simulink model "EnergyEstimationCorrection"  (R2020a)
settings: Solver=FixedStepAuto  StartTime=0  StopTime=time.Time(length(time.Time))  FixedStep=0.10  MaxStep=0.04  RelTol=1e-3
model workspace (MAT data in the model file):
  displayStatus = 1
values from neighbouring files (symbols this model uses):
  routeInfo = 4011    [EnergyEstimationMain.m]
  trip = tripUpdate    [EnergyEstimationMain.m]
undefined symbols (not defined in the file or in its folder): EbatRoute, EdriveRoute, energyDriveActual, energyDriveTrip, energyDriveTripCurrent, eState, massEstimate, sRoute, start, startRoute, stop, stopRoute, timeRoute, vehicleInfo, y, y_Estimate
libraries: simulink x1
(part 1 of 2)
settings Model: Creator=20184719  LastModifiedBy=20184719
settings OptimizationCC: ZeroExternalMemoryAtStartup=off  ZeroInternalMemoryAtStartup=off
settings DebuggingCC: UnderSpecifiedDimensionMsg=warning
settings HardwareCC: ProdBitPerPointer=32  ProdBitPerSizeT=32  ProdBitPerPtrDiffT=32  ProdLargestAtomicInteger=Long  ProdWordSize=32  ProdHWDeviceType=ARM Compatible->ARM 10
settings RTWCC: GenCodeOnly=on  TargetLang=C++
settings GRTTargetCC: TargetLangStandard=C++03 (ISO)  MatFileLogging=off  MultiInstanceERTCode=on  CodeInterfacePackaging=C++ class  MultiInstanceErrorCode=Warning

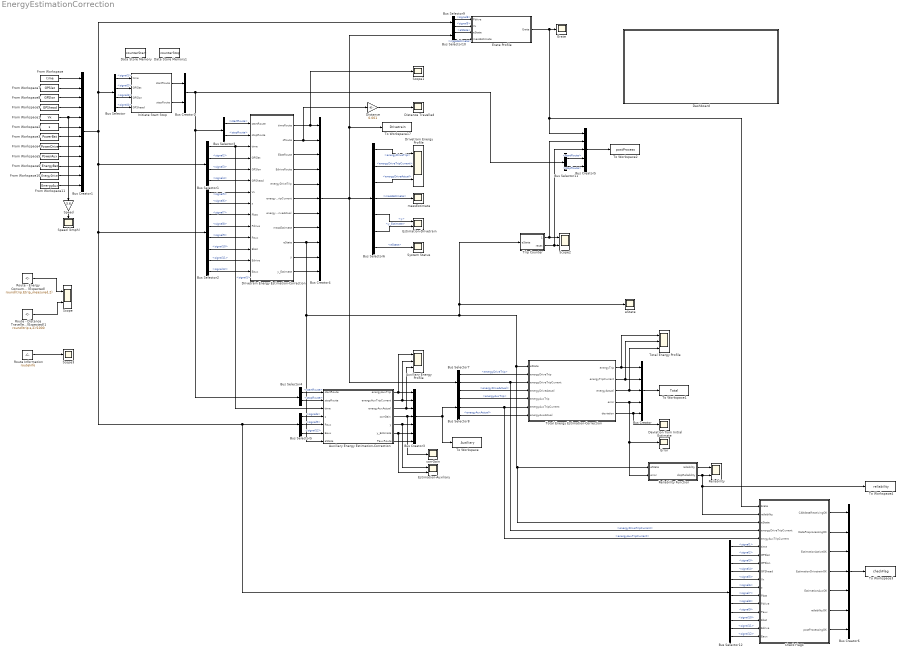
== system EnergyEstimationCorrection ==
  Auxiliary Energy Estimation-Correction : MATLAB Function  TreatAsAtomicUnit=on
  Auxiliary Energy Profile : Scope  NumInputPorts=3
  Bus Creator : BusCreator  Inputs=5
  Bus Creator1 : BusCreator  Inputs=12
  Bus Creator2 : BusCreator  Inputs=startRoute,stopRoute
  Bus Creator3 : BusCreator  Inputs=7
  Bus Creator4 : BusCreator  Inputs=timeRoute,sRoute,EbatRoute,EdriveRoute,energyDriveTrip,energyDriveTripCurrent,energyDriveActual,massEstimate,eState,y,y_Estimate
  Bus Creator5 : BusCreator  Inputs=5
  Bus Creator6 : BusCreator  Inputs=7
  Bus Selector : BusSelector  OutputSignals=signal1,signal2,signal3,signal4
  Bus Selector1 : BusSelector  OutputSignals=signal1,signal2,signal3,signal4
  Bus Selector10 : BusSelector  OutputSignals=eState,massEstimate
  Bus Selector11 : BusSelector  OutputSignals=startRoute,stopRoute
  Bus Selector12 : BusSelector  OutputSignals=signal1,signal2,signal3,signal4,signal5,signal6,signal7,signal8,signal9,signal10,signal11,signal12
  Bus Selector2 : BusSelector  OutputSignals=signal5,signal6,signal7,signal8,signal9,signal10,signal11,signal12
  Bus Selector3 : BusSelector  OutputSignals=startRoute,stopRoute
  Bus Selector4 : BusSelector  OutputSignals=startRoute,stopRoute
  Bus Selector5 : BusSelector  OutputSignals=signal6,signal9,signal12
  Bus Selector6 : BusSelector  OutputSignals=energyDriveTrip,energyDriveTripCurrent,energyDriveActual,massEstimate,y,y_Estimate,eState
  Bus Selector7 : BusSelector  OutputSignals=energyDriveTrip,energyDriveTripCurrent,energyDriveActual
  Bus Selector8 : BusSelector  OutputSignals=energyAuxTrip,energyAuxTripCurrent,energyAuxActual
  Bus Selector9 : BusSelector  OutputSignals=signal8,signal5
  Check Flags : MATLAB Function  TreatAsAtomicUnit=on
  Dashboard : Subsystem
  Data Store Memory : DataStoreMemory  DataStoreName=counterStart  ReadBeforeWriteMsg=warning  WriteAfterWriteMsg=warning  WriteAfterReadMsg=warning  ShowAdditionalParam=off  OutDataTypeStr=double
  Data Store Memory1 : DataStoreMemory  DataStoreName=counterStop  ReadBeforeWriteMsg=warning  WriteAfterWriteMsg=warning  WriteAfterReadMsg=warning  ShowAdditionalParam=off  OutDataTypeStr=double
  Deviation from Initial Estimate : Scope
  Distance : Gain  Gain=0.001
  Distance Travelled : Scope
  Drivetrain Energy Estimation-Correction : MATLAB Function  TreatAsAtomicUnit=on
  Drivetrain Energy Profile : Scope  NumInputPorts=3
  Erate : Scope
  Erate Profile : MATLAB Function  TreatAsAtomicUnit=on
  Error : Scope
  Estimation-Auxiliary : Scope  NumInputPorts=2
  Estimation-Drivetrain : Scope  NumInputPorts=2
  From Workspace : FromWorkspace  VariableName=time
  From Workspace1 : FromWorkspace  VariableName=Vx
  From Workspace10 : FromWorkspace  VariableName=EnergyDrive
  From Workspace11 : FromWorkspace  VariableName=EnergyAux
  From Workspace2 : FromWorkspace  VariableName=s
  From Workspace3 : FromWorkspace  VariableName=PowerBat
  From Workspace4 : FromWorkspace  VariableName=PowerDrive
  From Workspace5 : FromWorkspace  VariableName=PowerAux
  From Workspace6 : FromWorkspace  VariableName=EnergyBat
  From Workspace7 : FromWorkspace  VariableName=GPSlat
  From Workspace8 : FromWorkspace  VariableName=GPSlon
  From Workspace9 : FromWorkspace  VariableName=GPShead
  Initiate Start Stop : MATLAB Function  TreatAsAtomicUnit=on
  Reliability : Scope  NumInputPorts=2
  Reliability Function : MATLAB Function  TreatAsAtomicUnit=on
  Route - Distance Travelled (Expected)1 : Constant  Value=round(trip.s,2)/1000
  Route - Energy Consumption (Expected) : Constant  Value=round(trip.Etrip_measured,2)
  Route Information : Constant  Value=routeInfo
  Scope : Scope  NumInputPorts=2
  Scope1 : Scope
  Scope2 : Scope  NumInputPorts=2
  Scope3 : Scope
  Speed : Gain  Gain=3.6
  Speed (kmph) : Scope
  System Status : Scope
  To Workspace : ToWorkspace  VariableName=Auxiliary  SaveFormat=Timeseries  SampleTime=-1
  To Workspace1 : ToWorkspace  VariableName=Total  SaveFormat=Timeseries  SampleTime=-1
  To Workspace17 : ToWorkspace  VariableName=Drivetrain  SaveFormat=Timeseries  SampleTime=-1
  To Workspace2 : ToWorkspace  VariableName=postProcess  SaveFormat=Timeseries  SampleTime=-1
  To Workspace3 : ToWorkspace  VariableName=checkFlag  SaveFormat=Timeseries  SampleTime=-1
  To Workspace4 : ToWorkspace  VariableName=reliability  SaveFormat=Timeseries  SampleTime=-1
  Total Energy Estimation-Correction : MATLAB Function  TreatAsAtomicUnit=on
  Total Energy Profile : Scope  NumInputPorts=3
  Trip Counter : MATLAB Function  TreatAsAtomicUnit=on
  corrGain : Scope
  eState : Scope
  massEstimate : Scope
  wires:
  Drivetrain Energy Estimation-Correction/9(eState) -> Total Energy Estimation-Correction/1(eState), Check Flags/3(eState), Reliability Function/1(eState), Trip Counter/1(eState), eState/1, Auxiliary Energy Estimation-Correction/7(eState), Bus Creator4/9
  Bus Selector/1 -> Initiate Start Stop/1(time)  "<signal1>"
  Bus Selector/2 -> Initiate Start Stop/2(GPSlat)  "<signal2>"
  Bus Selector/3 -> Initiate Start Stop/3(GPSlon)  "<signal3>"
  Bus Selector/4 -> Initiate Start Stop/4(GPShead)  "<signal4>"
  Bus Selector1/1 -> Auxiliary Energy Estimation-Correction/3(time), Drivetrain Energy Estimation-Correction/3(time)  "<signal1>"
  Bus Selector1/2 -> Drivetrain Energy Estimation-Correction/4(GPSlat)  "<signal2>"
  Bus Selector1/3 -> Drivetrain Energy Estimation-Correction/5(GPSlon)  "<signal3>"
  Bus Selector1/4 -> Drivetrain Energy Estimation-Correction/6(GPShead)  "<signal4>"
  Bus Selector2/1 -> Drivetrain Energy Estimation-Correction/7(Vx)  "<signal5>"
  Bus Selector2/2 -> Drivetrain Energy Estimation-Correction/8(s)  "<signal6>"
  Bus Selector2/3 -> Drivetrain Energy Estimation-Correction/9(Pbat)  "<signal7>"
  Bus Selector2/4 -> Drivetrain Energy Estimation-Correction/10(Pdrive)  "<signal8>"
  Bus Selector2/5 -> Drivetrain Energy Estimation-Correction/11(Paux)  "<signal9>"
  Bus Selector2/6 -> Drivetrain Energy Estimation-Correction/12(Ebat)  "<signal10>"
  Bus Selector2/7 -> Drivetrain Energy Estimation-Correction/13(Edrive)  "<signal11>"
  Bus Selector2/8 -> Drivetrain Energy Estimation-Correction/14(Eaux)  "<signal12>"
  Initiate Start Stop/1(startRoute) -> Bus Creator2/1
  Initiate Start Stop/2(stopRoute) -> Bus Creator2/2
  Bus Creator2/1 -> Bus Selector4/1, Bus Selector3/1, Bus Selector11/1
  Bus Selector3/1 -> Drivetrain Energy Estimation-Correction/1(startRoute)  "<startRoute>"
  Bus Selector3/2 -> Drivetrain Energy Estimation-Correction/2(stopRoute)  "<stopRoute>"
  Bus Selector4/2 -> Auxiliary Energy Estimation-Correction/2(stopRoute)  "<stopRoute>"
  Bus Selector4/1 -> Auxiliary Energy Estimation-Correction/1(startRoute)  "<startRoute>"
  Bus Selector5/2 -> Auxiliary Energy Estimation-Correction/5(Paux)  "<signal9>"
  Bus Selector5/1 -> Auxiliary Energy Estimation-Correction/4(s)  "<signal6>"
  Bus Selector5/3 -> Auxiliary Energy Estimation-Correction/6(Eaux)  "<signal12>"
  Auxiliary Energy Estimation-Correction/1(energyAuxTrip) -> Bus Creator3/1, Auxiliary Energy Profile/1
  Auxiliary Energy Estimation-Correction/2(energyAuxTripCurrent) -> Bus Creator3/2, Auxiliary Energy Profile/2
  Auxiliary Energy Estimation-Correction/3(energyAuxActual) -> Bus Creator3/3, Auxiliary Energy Profile/3
  Auxiliary Energy Estimation-Correction/4(corrGain) -> corrGain/1, Bus Creator3/4
  Auxiliary Energy Estimation-Correction/5(y) -> Estimation-Auxiliary/1, Bus Creator3/5
  Auxiliary Energy Estimation-Correction/6(y_Estimate) -> Estimation-Auxiliary/2, Bus Creator3/6
  Drivetrain Energy Estimation-Correction/1(timeRoute) -> Scope1/1, Bus Creator4/1
  Drivetrain Energy Estimation-Correction/2(sRoute) -> Distance/1, Bus Creator4/2
  Drivetrain Energy Estimation-Correction/3(EbatRoute) -> Bus Creator4/3
  Drivetrain Energy Estimation-Correction/4(EdriveRoute) -> Bus Creator4/4
  Drivetrain Energy Estimation-Correction/5(energyDriveTrip) -> Bus Creator4/5
  Drivetrain Energy Estimation-Correction/6(energyDriveTripCurrent) -> Bus Creator4/6
  Drivetrain Energy Estimation-Correction/7(energyDriveActual) -> Bus Creator4/7
  Drivetrain Energy Estimation-Correction/8(massEstimate) -> Bus Creator4/8
  Drivetrain Energy Estimation-Correction/10(y) -> Bus Creator4/10
  Drivetrain Energy Estimation-Correction/11(y_Estimate) -> Bus Creator4/11
  Bus Creator4/1 -> Bus Selector10/1, To Workspace17/1, Bus Selector7/1, Bus Selector6/1
  Bus Selector6/2 -> Drivetrain Energy Profile/2  "<energyDriveTripCurrent>"
  Bus Selector6/1 -> Drivetrain Energy Profile/1  "<energyDriveTrip>"
  Bus Selector6/3 -> Drivetrain Energy Profile/3  "<energyDriveActual>"
  Bus Selector6/4 -> massEstimate/1  "<massEstimate>"
  Bus Selector6/5 -> Estimation-Drivetrain/1  "<y>"
  Bus Selector6/6 -> Estimation-Drivetrain/2  "<y_Estimate>"
  Bus Selector6/7 -> System Status/1  "<eState>"
  Bus Selector7/1 -> Total Energy Estimation-Correction/2(energyDriveTrip)  "<energyDriveTrip>"
  Bus Selector7/2 -> Check Flags/4(energyDriveTripCurrent), Total Energy Estimation-Correction/3(energyDriveTripCurrent)  "<energyDriveTripCurrent>"
  Bus Selector7/3 -> Total Energy Estimation-Correction/4(energyDriveActual)  "<energyDriveActual>"
  Bus Selector8/1 -> Total Energy Estimation-Correction/5(energyAuxTrip)  "<energyAuxTrip>"
  Bus Selector8/2 -> Check Flags/5(enrgyAuxTripCurrent), Total Energy Estimation-Correction/6(energyAuxTripCurrent)  "<energyAuxTripCurrent>"
  Bus Selector8/3 -> Total Energy Estimation-Correction/7(energyAuxActual)  "<energyAuxActual>"
  Bus Creator3/1 -> To Workspace/1, Bus Selector8/1
  From Workspace/1 -> Bus Creator1/1
  Bus Creator1/1 -> Bus Selector9/1, Bus Selector/1, Bus Selector1/1, Bus Selector2/1, Bus Selector12/1, Bus Selector5/1
  From Workspace7/1 -> Bus Creator1/2
  From Workspace8/1 -> Bus Creator1/3
  From Workspace9/1 -> Bus Creator1/4
  From Workspace1/1 -> Bus Creator1/5, Speed/1
  From Workspace2/1 -> Bus Creator1/6
  From Workspace3/1 -> Bus Creator1/7
  From Workspace4/1 -> Bus Creator1/8
  From Workspace5/1 -> Bus Creator1/9
  From Workspace6/1 -> Bus Creator1/10
  From Workspace10/1 -> Bus Creator1/11
  From Workspace11/1 -> Bus Creator1/12
  Total Energy Estimation-Correction/1(energyTrip) -> Bus Creator/1, Total Energy Profile/1
  Total Energy Estimation-Correction/2(energyTripCurrent) -> Bus Creator/2, Total Energy Profile/2
  Total Energy Estimation-Correction/3(energyActual) -> Bus Creator/3, Total Energy Profile/3
  Total Energy Estimation-Correction/4(error) -> Reliability Function/2(error), Error/1, Bus Creator/4
  Bus Creator/1 -> To Workspace1/1
  Speed/1 -> Speed (kmph)/1
  Route - Energy Consumption (Expected)/1 -> Scope/1
  Route - Distance Travelled (Expected)1/1 -> Scope/2
  Distance/1 -> Distance Travelled/1
  Total Energy Estimation-Correction/5(deviation) -> Deviation from Initial Estimate/1, Bus Creator/5
  Reliability Function/1(reliability) -> Reliability/1
  Reliability Function/2(dispReliability) -> Check Flags/2(reliability), To Workspace4/1, Reliability/2
  Erate Profile/1(Erate) -> Check Flags/1(Erate), Bus Creator5/1, Erate/1
  Bus Selector9/1 -> Erate Profile/1(Pdrive)  "<signal8>"
  Bus Selector9/2 -> Erate Profile/2(Vx)  "<signal5>"
  Bus Selector10/1 -> Erate Profile/3(eState)  "<eState>"
  Bus Selector10/2 -> Erate Profile/4(massEstimate)  "<massEstimate>"
  Trip Counter/1(counter) -> Bus Creator5/2, Scope2/1
  Trip Counter/2(reset) -> Bus Creator5/3, Scope2/2
  Bus Creator5/1 -> To Workspace2/1
  Auxiliary Energy Estimation-Correction/7(PauxRoute) -> Bus Creator3/7
  Bus Selector11/1 -> Bus Creator5/4  "<startRoute>"
  Bus Selector11/2 -> Bus Creator5/5  "<stopRoute>"
  Route Information/1 -> Scope3/1
  Bus Selector12/1 -> Check Flags/6(time)  "<signal1>"
  Bus Selector12/2 -> Check Flags/7(GPSlat)  "<signal2>"
  Bus Selector12/3 -> Check Flags/8(GPSlon)  "<signal3>"
  Bus Selector12/4 -> Check Flags/9(GPShead)  "<signal4>"
  Bus Selector12/5 -> Check Flags/10(Vx)  "<signal5>"
  Bus Selector12/6 -> Check Flags/11(s)  "<signal6>"
  Bus Selector12/7 -> Check Flags/12(Pbat)  "<signal7>"
  Bus Selector12/8 -> Check Flags/13(Pdrive)  "<signal8>"
  Bus Selector12/9 -> Check Flags/14(Paux)  "<signal9>"
  Bus Selector12/10 -> Check Flags/15(Ebat)  "<signal10>"
  Bus Selector12/11 -> Check Flags/16(Edrive)  "<signal11>"
  Bus Selector12/12 -> Check Flags/17(Eaux)  "<signal12>"
  Check Flags/7(postProcessingOK) -> Bus Creator6/7
  Check Flags/6(reliabilityOK) -> Bus Creator6/6
  Check Flags/5(EstimationAuxOK) -> Bus Creator6/5
  Check Flags/4(EstimationDrivetrainOK) -> Bus Creator6/4
  Check Flags/3(EstimationActiveOK) -> Bus Creator6/3
  Check Flags/2(DataPreprocessingOK) -> Bus Creator6/2
  Check Flags/1(CANdataReceivingOK) -> Bus Creator6/1
  Bus Creator6/1 -> To Workspace3/1

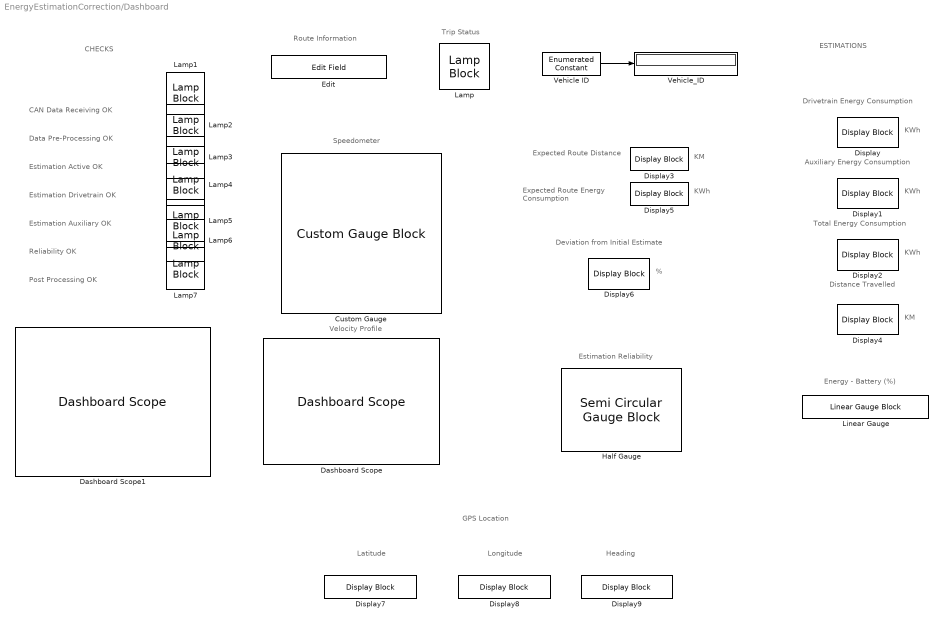
== system EnergyEstimationCorrection/Dashboard ==
  note: Energy - Battery (%)
  note: Trip Status
  note: Route Information
  note: Speedometer
  note: Velocity Profile
  note: Drivetrain Energy Consumption
  note: Auxiliary Energy Consumption
  note: Total Energy Consumption
  note: Expected Route
      | Distance
  note: Expected Route
      | Energy Consumption
  note: KM
  note: KWh
  note: Distance Travelled
  note: KM
  note: KWh
  note: KWh
  note: KWh
  note: Estimation Reliability
  note: Deviation from Initial Estimate
  note: %
  note: CAN Data Receiving OK
  note: CHECKS
  note: ESTIMATIONS
  note: Data Pre-Processing OK
  note: Estimation Active OK
  note: Estimation Drivetrain OK
  note: Estimation Auxiliary OK
  note: Reliability OK
  note: Post Processing OK
  note: Latitude
  note: Longitude
  note: Heading
  note: GPS Location
  Custom Gauge : CustomGaugeBlock  NeedleImage=data:image/svg+xml;base64,PD94bWwgdmVyc2lvbj0iMS4wIiBlbmNvZGluZz0idXRmLTgiPz4KPCEtLSBHZW5lcmF0b3I6IEFkb2JlIElsbHVzdHJhdG9yIDE5LjIuMSwgU1ZHIEV4cG9ydCBQbHVnLUluIC4gU1ZHIFZlcnNpb246IDYuMDAgQnVpbGQgMCkgIC0tPgo8c3ZnIHZlcnNpb249IjEuMSIgeG1sbnM9Imh0dHA6Ly93d3cudzMub3JnLzIwMDAvc3ZnIiB4bWxuczp4bGluaz0iaHR0cDovL3d3dy53My5vcmcvMTk5OS94bGluayIgeD0iMHB4IiB5PSIwcHgiCgkgdmlld0JveD0iMCAwIDIwMCA1MCIgc3R5bGU9ImVuYWJsZS1iYWNrZ3JvdW5kOm5ldyAw ...(+9940 chars)  NeedleXPos=0.39639858870118533  NeedleYPos=0.48371466282014003  NeedleHeight=0.10035881361873647  NeedleWidth=0.16533373475036106  NeedleInitialRotation=-59.94322499147643  BackgroundImage=data:image/svg+xml;base64,PD94bWwgdmVyc2lvbj0iMS4wIiBlbmNvZGluZz0iVVRGLTgiIHN0YW5kYWxvbmU9Im5vIj8+CjwhLS0gR2VuZXJhdG9yOiBBZG9iZSBJbGx1c3RyYXRvciAxOS4yLjEsIFNWRyBFeHBvcnQgUGx1Zy1JbiAuIFNWRyBWZXJzaW9uOiA2LjAwIEJ1aWxkIDApICAtLT4KCjxzdmcKICAgeG1sbnM6ZGM9Imh0dHA6Ly9wdXJsLm9yZy9kYy9lbGVtZW50cy8xLjEvIgogICB4bWxuczpjYz0iaHR0cDovL2NyZWF0aXZlY29tbW9ucy5vcmcvbnMjIgogICB4bWxuczpyZGY9Imh0dHA6Ly93d3cudzMub3JnLzE5OTkvMDIvMjItcmRmLXN5bnRh ...(+9660 chars)  GaugeMax=80  GaugeArcDefined=true  GaugeArcRadius=0.117516010929013  GaugeArcStrokeWidth=0.034366217970160734  GaugeArcRotation=240.5385250290321  GaugeArcRatio=0.8333333333333  GaugeArcTransparency=0.3739565943238731  ValueArcTransparency=0.5021702838063439  ValueArcColor=#40b0ac  GaugeTickColor=#faf5c8  ScaleColorsJSON=[]  fixedAspectRatio=on  IsLinearGauge=false  GaugeTrackLeft=0.35  GaugeTrackTop=0.35  GaugeTrackHeight=0.1  GaugeTrackWidth=0.3  GaugeTrackRotation=0
  Dashboard Scope : DashboardScope  Ymin=0  Ymax=80
  Dashboard Scope1 : DashboardScope  Ymin=-1  Ymax=15  ScaleAtStop=off
  Display{,1..9} (10 alike) : DisplayBlock  LabelPosition=Hide  Format=short  Transparency=1
  Edit : EditField  LabelPosition=Hide  ShowInitialText=on  Alignment=Center
  Half Gauge : SemiCircularGaugeBlock
  Lamp{,1..7} (8 alike) : LampBlock
  Linear Gauge : LinearGaugeBlock
  Vehicle ID : simulink/Sources/Enumerated Constant  OutDataTypeStr=Enum: vehicleInfo  Value=vehicleInfo.False  SampleTime=inf  mask(Enumerated Constant){}
      mask Display:
      | % This is a new mask on top of the base mask.
      | % Use "View base mask" link below to see the base mask.
      | disp(Vehicle - Info)
  Vehicle_ID : Display
  wires:
  Vehicle ID/1 -> Vehicle_ID/1

== matlab function EnergyEstimationCorrection/Reliability Function ==
  data: eState input; error input; reliability output; dispReliability output
function [reliability, dispReliability] = fcn(eState,error)

%   Author: Dhruv Jagga
%   Project: Source Code - Cloud Your Bus
%   email: d.jagga@tue.nl
%   Date: 10-12-2019;
%   Revised: 06-08-2020

if eState ==  1
    if abs(error) <= 20
        reliability = 100 - abs(error) * 5;
    else 
        reliability = 0;
    end
    
else
    reliability = 0;
end

if reliability > 95
    dispReliability = 100;
else
    dispReliability = reliability;
end
    
end

== matlab function EnergyEstimationCorrection/Auxiliary Energy Estimation-Correction ==
  data: energyAuxTrip output; energyAuxTripCurrent output; energyAuxActual output; corrGain output; startRoute input; y output; stopRoute input; time input; s input; Paux input; Eaux input; eState input; y_Estimate output; trip parameter; PauxRoute output
function [energyAuxTrip,energyAuxTripCurrent,energyAuxActual,corrGain,y,y_Estimate, PauxRoute] = fcn(startRoute,stopRoute,time,s,Paux,Eaux,eState,trip)

%   Author: Dhruv Jagga
%   Project: Source Code - Cloud Your Bus
%   email: d.jagga@tue.nl
%   Date: 10-12-2019;
%   Revised: 06-08-2020

% Define and Initializing the variables
% Initiated as persistent variables for retaining values of these variables
% to be used in the next time cycle

persistent timeStamp sStamp EAuxStamp P corrGainPrev

if isempty(timeStamp)
    timeStamp = 0.0;
end

if isempty(sStamp)
    sStamp = 0.0;
end

if isempty(EAuxStamp)
    EAuxStamp = 0.0;
end

if isempty(P)
    P = eye(1);
end

if isempty(corrGainPrev)
    corrGainPrev = 0.1;
end

%%%%%%%%%%%%%%%%%%%%%%%%%%%%%%%%%%%%%%%%%%%%%%%%%%%%%%%%%%%%%%%%%%%%%%%%%%%%%%%%%%%%%%%%%%%%%%%%%%
% Variable time stamp resetting

if startRoute == true && stopRoute == false
    timeStamp = time;
    sStamp = s;
    EAuxStamp = Eaux;
end

%%%%%%%%%%%%%%%%%%%%%%%%%%%%%%%%%%%%%%%%%%%%%%%%%%%%%%%%%%%%%%%%%%%%%%%%%%%%%%%%%%%%%%%%%%%%%%%%%%
%%%%%%%%%%%%%%%%%%%%%%%%%%%%%%%%%%%%%%%%%%%%%%%%%%%%%%%%%%%%%%%%%%%%%%%%%%%%%%%%%%%%%%%%%%%%%%%%%%

% Switch to new state based upon value state register
if  eState == 0                        % State when the trip has not yet started
    energyAuxTrip= 0;
    energyAuxTripCurrent = 0;
    energyAuxActual= 0;
    corrGain = 0;
    y = 0;
    y_Estimate = 0;
    
    %%%%%%%%%%%%%%%%%%%%%%%%%%%%%%%%%%%%%%%%%%%%%%%%%%%%%%%%%%%%%%%%%%%%%%%%%%%%%%%%%%%%%%%%%%%%%%%%%%
    
elseif  eState == 1                        % State when the trip has started
    timeRoute = time - timeStamp;
    sRoute    = s - sStamp;
    EAuxRoute = Eaux - EAuxStamp;
    
    % Energy estimate Auxillary
    EuseAuxEstimate  = cumsum(trip.Paux)*corrGainPrev/3.6e6;    % Energy estimate in KWh
    EuseAuxFinal = EuseAuxEstimate(length(EuseAuxEstimate));
%     EuseAuxCurrent = interp1(trip.timeAux,EuseAuxEstimate,timeRoute);                     % Energy estimate in KWh
    EuseAuxCurrent = interp1(trip.sRoute,EuseAuxEstimate,sRoute);                     % Energy estimate in KWh
    
    % Total energy consumption estimate for the entire trip
    energyAuxTrip = EuseAuxFinal;                               % Energy consumtion Estimate given at the start of the trip for entire route
    energyAuxTripCurrent = EuseAuxCurrent;
    
    % Actual energy consumption
    energyAuxActual = EAuxRoute;                                       % Actual total ennergy consumed over the trip
    
    %%%%%%%%%%%%%%%%%%%%%%%%%%%%%%%%%%%%%%%%%%%%%%%%%%%%%%%%%%%%%%%%%%%%%%%%%%%%%%%%%%%%%%%%%%%%%%%%%%  
    
    % METHOD 4 - MASS ESTIMATE (Kalman Filter Approach)
    
    y = EAuxRoute;
    
    phi = cumsum(trip.Paux)/3.6e6;
    phi = phi';
    
    yEstimate = phi'*corrGainPrev;
    yEstimate = interp1(trip.sRoute,yEstimate,sRoute);
    
    y_Estimate = yEstimate;
    
    for i = 1:length(trip.Paux)
        R1 = 1e-5;
        R2 = 1;
        pPrev = P;
        
        P = pPrev + R1 - ((pPrev*(phi(i)*phi(i)')*pPrev)/(R2 + (phi(i)'*pPrev*phi(i))));
        Q = pPrev/(R2 + (phi(i)'*pPrev*phi(i)));
        
        K = Q * phi(i);
    end
    
    if sRoute > 100
        corrGain = corrGainPrev + K * (y - yEstimate);
    else
        corrGain = 0.1;
    end
    
    corrGainPrev = corrGain;

else
    energyAuxTrip= 0;
    energyAuxTripCurrent = 0;
    energyAuxActual= 0;
    corrGain = 0;
    y = 0;
    y_Estimate = 0;
    
end

% Storing Auxiliary Power for post processing and database update

if eState == 1
    PauxRoute = Paux;
else
    PauxRoute = 0;
end
end

== matlab function EnergyEstimationCorrection/Total Energy Estimation-Correction ==
  data: eState input; energyTrip output; energyTripCurrent output; energyActual output; energyDriveTrip input; energyDriveTripCurrent input; energyDriveActual input; energyAuxTrip input; energyAuxTripCurrent input; energyAuxActual input; trip parameter; error output; deviation output
function [energyTrip,energyTripCurrent,energyActual,error,deviation] = fcn(eState,energyDriveTrip,energyDriveTripCurrent,energyDriveActual,energyAuxTrip,energyAuxTripCurrent,energyAuxActual,trip)

%   Author: Dhruv Jagga
%   Project: Source Code - Cloud Your Bus
%   email: d.jagga@tue.nl
%   Date: 10-12-2019;
%   Revised: 06-08-2020

if eState == 1
    energyTrip = energyDriveTrip + energyAuxTrip;                               % Energy consumtion Estimate given at the start of the trip for entire route
    energyTripCurrent = energyDriveTripCurrent + energyAuxTripCurrent;
    
%     if isnan(energyTrip) || isnan(energyTripCurrent)
%         energyTrip = 0;
%         energyTripCurrent = 0;
%     end
    
    % Actual energy consumption
    energyActual = energyDriveActual + energyAuxActual;
    
    %%%%%%%%%%%%%%%%%%%%%%%%%%%%%%%%%%%%%%%%%%%%%%%%%%%%%%%%%%%%%%%%%%%%%%%%%%%%%%%%%%%%%%%%%%%%%%%%%%
    % Error Calculation between actual and estimated energy.
    
    deviation =(energyTrip - trip.Etrip_measured)/trip.Etrip_measured * 100;
    
    error = (energyTripCurrent - energyActual)/energyActual * 100;
    
%     if abs(deviation) > 50
%         deviation = 0;
%     else
%         deviation = deviation;
%     end
    
else eState == 0
    energyTrip          = 0;
    energyTripCurrent   = 0;
    energyActual        = 0;
    error               = 0;
    deviation           = 0;
    
end
end

== matlab function EnergyEstimationCorrection/Erate Profile ==
  data: Pdrive input; Erate output; Vx input; eState input; massEstimate input
function Erate = ErateProfile(Pdrive,Vx,eState,massEstimate)

%   Author: Dhruv Jagga
%   Project: Source Code - Cloud Your Bus
%   email: d.jagga@tue.nl
%   Date: 10-12-2019;
%   Revised: 06-08-2020

if eState == 1
    
    if Vx == 0
        ForceDrive = 0;
        Erate = ForceDrive/massEstimate;
    else
        ForceDrive = Pdrive/Vx;
        Erate = ForceDrive/massEstimate;
    end
     
else eState == 0
    Erate = 0;
end


end

== matlab function EnergyEstimationCorrection/Trip Counter ==
  data: eState input; counter output; reset output
function [counter,reset] = fcn(eState)

%   Author: Dhruv Jagga
%   Project: Source Code - Cloud Your Bus
%   email: d.jagga@tue.nl
%   Date: 10-12-2019;
%   Revised: 06-08-2020

persistent count previouseState reset1

if isempty(count)
    count = 0;
end

if isempty(reset1)
    reset1 = 0;
end

if isempty(previouseState)
    previouseState = 0;
end

if eState ~= previouseState
    if eState == 1
        count = count + 1;
    else
        count = count;
    end
end


if count == 3
    count = 1;
    reset1 = reset1 + 1;
else
    reset1 = reset1;
end

previouseState = eState;

counter = count;
reset = reset1;

end

== matlab function EnergyEstimationCorrection/Check Flags ==
  data: Erate input; reliability input; eState input; energyDriveTripCurrent input; enrgyAuxTripCurrent input; time input; CANdataReceivingOK output; GPSlat input; GPSlon input; GPShead input; Vx input; s input; Pbat input; Pdrive input; Paux input; Ebat input; Edrive input; Eaux input; DataPreprocessingOK output; EstimationActiveOK output; EstimationDrivetrainOK output; EstimationAuxOK output; reliabilityOK output; postProcessingOK output
function [CANdataReceivingOK,DataPreprocessingOK,EstimationActiveOK,EstimationDrivetrainOK,EstimationAuxOK,reliabilityOK,postProcessingOK]  = checkFlagFunc(Erate,reliability,eState,energyDriveTripCurrent,enrgyAuxTripCurrent,time,GPSlat,GPSlon,GPShead,Vx,s,Pbat,Pdrive,Paux,Ebat,Edrive,Eaux)

%   Author: Dhruv Jagga
%   Project: Source Code - Cloud Your Bus
%   email: d.jagga@tue.nl
%   Date: 10-12-2019;
%   Revised: 06-08-2020

if ~isnan(time) && ~isnan(GPSlat) && ~isnan(GPSlon) && ~isnan(GPShead) && ~isnan(Vx)
    CANdataReceivingOK = true;
else
    CANdataReceivingOK = false;
end

if ~isnan(s) && ~isnan(Pbat) && ~isnan(Pdrive) && ~isnan(Paux) && ~isnan(Ebat) && ~isnan(Edrive) && ~isnan(Eaux)
    DataPreprocessingOK = true;
else
    DataPreprocessingOK = false;
end

if eState == 1
    EstimationActiveOK = true;
else
    EstimationActiveOK = false;
end

if eState == 1 && energyDriveTripCurrent > 0 && ~isnan(energyDriveTripCurrent)
    EstimationDrivetrainOK = true;
else
    EstimationDrivetrainOK = false;
end

if eState == 1 && enrgyAuxTripCurrent > 0 && ~isnan(enrgyAuxTripCurrent)
    EstimationAuxOK = true;
else
    EstimationAuxOK = false;
end
    
if eState == 1 && reliability > 0 && ~isnan(reliability)
    reliabilityOK = true;
else
    reliabilityOK = false;
end

if eState == 1 && ~isnan(Erate)
    postProcessingOK = true;
else
    postProcessingOK = false;
end

end
